simulink model "figure_2_7"  (R2026a)
settings: Solver=ode5  FixedStep=1e-4
settings Model: Creator=yagmu  LastModifiedBy=yagmu

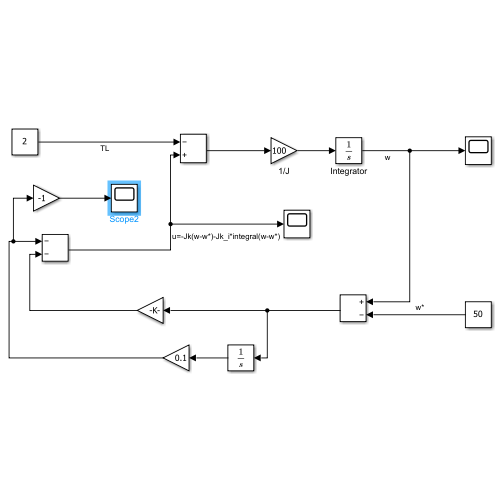
[thumbnail: Simulink's stored preview of the top-level diagram]
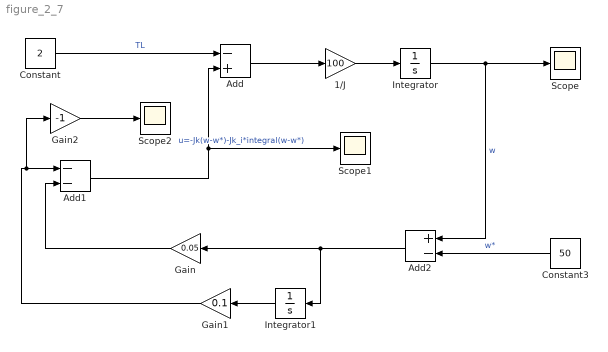
== system figure_2_7 ==
  1/J : Gain  Gain=100
  Add : Sum  Inputs=-+
  Add1 : Sum  Inputs=--
  Add2 : Sum  Inputs=+-
  Constant : Constant  Value=2
  Constant3 : Constant  Value=50
  Gain : Gain  Gain=0.05
  Gain1 : Gain  Gain=0.1
  Gain2 : Gain  Gain=-1
  Integrator : Integrator  InitialCondition=50
  Integrator1 : Integrator
  Scope : Scope
      settings: ActiveDisplayYMinimum=19.555955292240327  ActiveDisplayYMaximum=53.902511940813639
  Scope1 : Scope
      settings: ActiveDisplayYMinimum=1.8875000000000441  ActiveDisplayYMaximum=2.0124999999996005
  Scope2 : Scope
      settings: ActiveDisplayYMinimum=-0.25433049667609031  ActiveDisplayYMaximum=2.2889744700848134  DataLoggingVariableName=ScopeData2
  wires:
  Add/1 -> 1/J/1
  1/J/1 -> Integrator/1
  Integrator/1 -> Add2/1, Scope/1  "w"
  Add1/1 -> Add/2, Scope1/1  "u=-Jk(w-w*)-Jk_i*integral(w-w*)"
  Constant3/1 -> Add2/2  "w*"
  Constant/1 -> Add/1  "TL"
  Integrator1/1 -> Gain1/1
  Add2/1 -> Integrator1/1, Gain/1
  Gain/1 -> Add1/2
  Gain1/1 -> Gain2/1, Add1/1
  Gain2/1 -> Scope2/1
